simulink model "Dynamic_Simulation"  (R2019a)
settings: Solver=VariableStepAuto  StartTime=0.0  StopTime=10.0  RelTol=1e-3
values from neighbouring files (symbols this model uses):
  Car = feval(Files.Car_File)    [Run_Program.m]
settings Model: Creator=Foster  LastModifiedBy=Foster

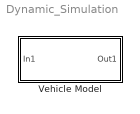
== system Dynamic_Simulation ==
  Vehicle Model : Subsystem

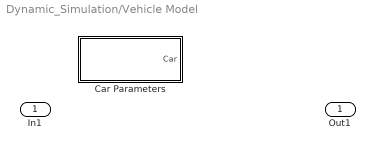
== system Dynamic_Simulation/Vehicle Model ==
  In1 : Inport
  Car Parameters : Subsystem
  Out1 : Outport

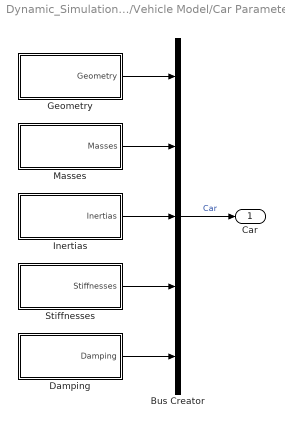
== system Dynamic_Simulation/Vehicle Model/Car Parameters ==
  Bus Creator : BusCreator  Inputs=5
  Damping : Subsystem
  Geometry : Subsystem
  Inertias : Subsystem
  Masses : Subsystem
  Stiffnesses : Subsystem
  Car : Outport
  wires:
  Geometry/1(Geometry) -> Bus Creator/1
  Masses/1(Masses) -> Bus Creator/2
  Inertias/1(Inertias) -> Bus Creator/3
  Stiffnesses/1(Stiffnesses) -> Bus Creator/4
  Damping/1(Damping) -> Bus Creator/5
  Bus Creator/1 -> Car/1  "Car"

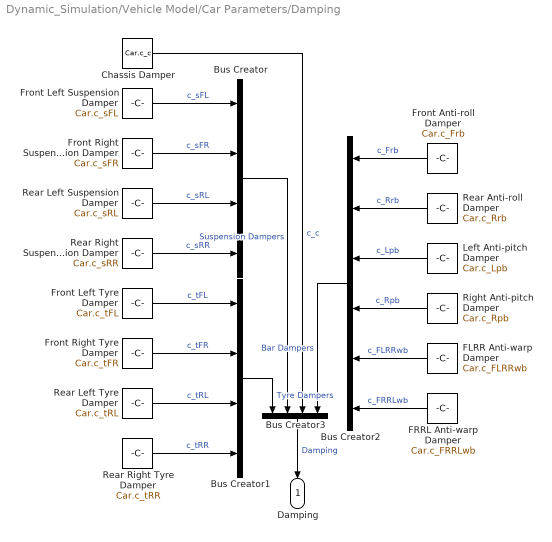
== system Dynamic_Simulation/Vehicle Model/Car Parameters/Damping ==
  Bus Creator : BusCreator  Inputs=4
  Bus Creator1 : BusCreator  Inputs=4
  Bus Creator2 : BusCreator  Inputs=6
  Bus Creator3 : BusCreator  Inputs=4
  Chassis Damper : Constant  Value=Car.c_c
  FLRR Anti-warp Damper : Constant  Value=Car.c_FLRRwb
  FRRL Anti-warp Damper : Constant  Value=Car.c_FRRLwb
  Front Anti-roll Damper : Constant  Value=Car.c_Frb
  Front Left Suspension Damper : Constant  Value=Car.c_sFL
  Front Left Tyre Damper : Constant  Value=Car.c_tFL
  Front Right Suspension Damper : Constant  Value=Car.c_sFR
  Front Right Tyre Damper : Constant  Value=Car.c_tFR
  Left Anti-pitch Damper : Constant  Value=Car.c_Lpb
  Rear Anti-roll Damper : Constant  Value=Car.c_Rrb
  Rear Left Suspension Damper : Constant  Value=Car.c_sRL
  Rear Left Tyre Damper : Constant  Value=Car.c_tRL
  Rear Right Suspension Damper : Constant  Value=Car.c_sRR
  Rear Right Tyre Damper : Constant  Value=Car.c_tRR
  Right Anti-pitch Damper : Constant  Value=Car.c_Rpb
  Damping : Outport
  wires:
  Front Left Suspension Damper/1 -> Bus Creator/1  "c_sFL"
  Front Right Suspension Damper/1 -> Bus Creator/2  "c_sFR"
  Rear Left Suspension Damper/1 -> Bus Creator/3  "c_sRL"
  Rear Right Suspension Damper/1 -> Bus Creator/4  "c_sRR"
  Front Left Tyre Damper/1 -> Bus Creator1/1  "c_tFL"
  Front Right Tyre Damper/1 -> Bus Creator1/2  "c_tFR"
  Rear Left Tyre Damper/1 -> Bus Creator1/3  "c_tRL"
  Rear Right Tyre Damper/1 -> Bus Creator1/4  "c_tRR"
  Chassis Damper/1 -> Bus Creator3/3  "c_c"
  Front Anti-roll Damper/1 -> Bus Creator2/1  "c_Frb"
  Rear Anti-roll Damper/1 -> Bus Creator2/2  "c_Rrb"
  Left Anti-pitch Damper/1 -> Bus Creator2/3  "c_Lpb"
  Right Anti-pitch Damper/1 -> Bus Creator2/4  "c_Rpb"
  FLRR Anti-warp Damper/1 -> Bus Creator2/5  "c_FLRRwb"
  FRRL Anti-warp Damper/1 -> Bus Creator2/6  "c_FRRLwb"
  Bus Creator3/1 -> Damping/1  "Damping"
  Bus Creator1/1 -> Bus Creator3/1  "Tyre Dampers"
  Bus Creator/1 -> Bus Creator3/2  "Suspension Dampers"
  Bus Creator2/1 -> Bus Creator3/4  "Bar Dampers"

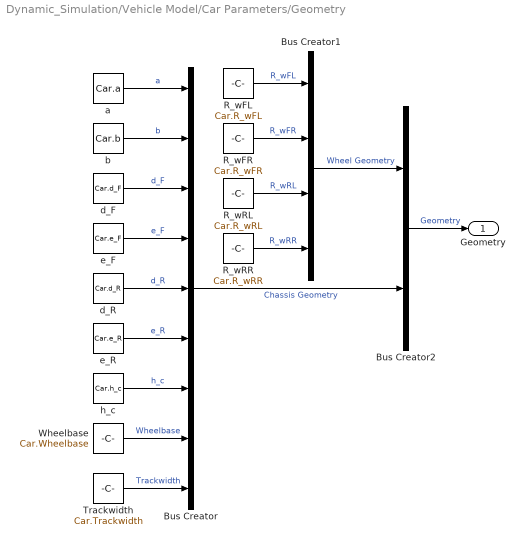
== system Dynamic_Simulation/Vehicle Model/Car Parameters/Geometry ==
  Bus Creator : BusCreator  Inputs=9
  Bus Creator1 : BusCreator  Inputs=4
  Bus Creator2 : BusCreator  Inputs=2
  R_wFL : Constant  Value=Car.R_wFL
  R_wFR : Constant  Value=Car.R_wFR
  R_wRL : Constant  Value=Car.R_wRL
  R_wRR : Constant  Value=Car.R_wRR
  Trackwidth : Constant  Value=Car.Trackwidth
  Wheelbase : Constant  Value=Car.Wheelbase
  a : Constant  Value=Car.a
  b : Constant  Value=Car.b
  d_F : Constant  Value=Car.d_F
  d_R : Constant  Value=Car.d_R
  e_F : Constant  Value=Car.e_F
  e_R : Constant  Value=Car.e_R
  h_c : Constant  Value=Car.h_c
  Geometry : Outport
  wires:
  a/1 -> Bus Creator/1  "a"
  b/1 -> Bus Creator/2  "b"
  d_F/1 -> Bus Creator/3  "d_F"
  e_F/1 -> Bus Creator/4  "e_F"
  d_R/1 -> Bus Creator/5  "d_R"
  e_R/1 -> Bus Creator/6  "e_R"
  Trackwidth/1 -> Bus Creator/9  "Trackwidth"
  Wheelbase/1 -> Bus Creator/8  "Wheelbase"
  h_c/1 -> Bus Creator/7  "h_c"
  R_wFL/1 -> Bus Creator1/1  "R_wFL"
  R_wFR/1 -> Bus Creator1/2  "R_wFR"
  R_wRL/1 -> Bus Creator1/3  "R_wRL"
  R_wRR/1 -> Bus Creator1/4  "R_wRR"
  Bus Creator/1 -> Bus Creator2/2  "Chassis Geometry"
  Bus Creator1/1 -> Bus Creator2/1  "Wheel Geometry"
  Bus Creator2/1 -> Geometry/1  "Geometry"

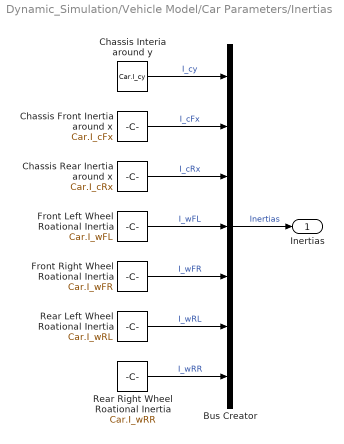
== system Dynamic_Simulation/Vehicle Model/Car Parameters/Inertias ==
  Bus Creator : BusCreator  Inputs=7
  Chassis Front Inertia around x : Constant  Value=Car.I_cFx
  Chassis Interia around y : Constant  Value=Car.I_cy
  Chassis Rear Inertia around x : Constant  Value=Car.I_cRx
  Front Left Wheel Roational Inertia : Constant  Value=Car.I_wFL
  Front Right Wheel Roational Inertia : Constant  Value=Car.I_wFR
  Rear Left Wheel Roational Inertia : Constant  Value=Car.I_wRL
  Rear Right Wheel Roational Inertia : Constant  Value=Car.I_wRR
  Inertias : Outport
  wires:
  Chassis Interia around y/1 -> Bus Creator/1  "I_cy"
  Chassis Front Inertia around x/1 -> Bus Creator/2  "I_cFx"
  Chassis Rear Inertia around x/1 -> Bus Creator/3  "I_cRx"
  Front Left Wheel Roational Inertia/1 -> Bus Creator/4  "I_wFL"
  Front Right Wheel Roational Inertia/1 -> Bus Creator/5  "I_wFR"
  Rear Left Wheel Roational Inertia/1 -> Bus Creator/6  "I_wRL"
  Rear Right Wheel Roational Inertia/1 -> Bus Creator/7  "I_wRR"
  Bus Creator/1 -> Inertias/1  "Inertias"

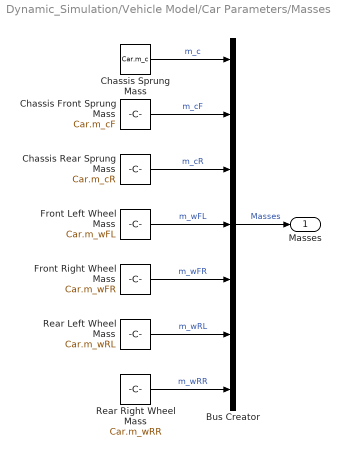
== system Dynamic_Simulation/Vehicle Model/Car Parameters/Masses ==
  Bus Creator : BusCreator  Inputs=7
  Chassis Front Sprung Mass : Constant  Value=Car.m_cF
  Chassis Rear Sprung Mass : Constant  Value=Car.m_cR
  Chassis Sprung Mass : Constant  Value=Car.m_c
  Front Left Wheel Mass : Constant  Value=Car.m_wFL
  Front Right Wheel Mass : Constant  Value=Car.m_wFR
  Rear Left Wheel Mass : Constant  Value=Car.m_wRL
  Rear Right Wheel Mass : Constant  Value=Car.m_wRR
  Masses : Outport
  wires:
  Chassis Sprung Mass/1 -> Bus Creator/1  "m_c"
  Chassis Front Sprung Mass/1 -> Bus Creator/2  "m_cF"
  Chassis Rear Sprung Mass/1 -> Bus Creator/3  "m_cR"
  Front Left Wheel Mass/1 -> Bus Creator/4  "m_wFL"
  Front Right Wheel Mass/1 -> Bus Creator/5  "m_wFR"
  Rear Left Wheel Mass/1 -> Bus Creator/6  "m_wRL"
  Rear Right Wheel Mass/1 -> Bus Creator/7  "m_wRR"
  Bus Creator/1 -> Masses/1  "Masses"

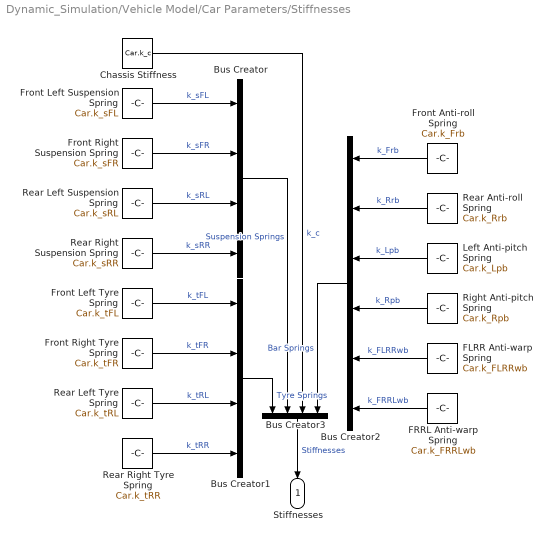
== system Dynamic_Simulation/Vehicle Model/Car Parameters/Stiffnesses ==
  Bus Creator : BusCreator  Inputs=4
  Bus Creator1 : BusCreator  Inputs=4
  Bus Creator2 : BusCreator  Inputs=6
  Bus Creator3 : BusCreator  Inputs=4
  Chassis Stiffness : Constant  Value=Car.k_c
  FLRR Anti-warp Spring : Constant  Value=Car.k_FLRRwb
  FRRL Anti-warp Spring : Constant  Value=Car.k_FRRLwb
  Front Anti-roll Spring : Constant  Value=Car.k_Frb
  Front Left Suspension Spring : Constant  Value=Car.k_sFL
  Front Left Tyre Spring : Constant  Value=Car.k_tFL
  Front Right Suspension Spring : Constant  Value=Car.k_sFR
  Front Right Tyre Spring : Constant  Value=Car.k_tFR
  Left Anti-pitch Spring : Constant  Value=Car.k_Lpb
  Rear Anti-roll Spring : Constant  Value=Car.k_Rrb
  Rear Left Suspension Spring : Constant  Value=Car.k_sRL
  Rear Left Tyre Spring : Constant  Value=Car.k_tRL
  Rear Right Suspension Spring : Constant  Value=Car.k_sRR
  Rear Right Tyre Spring : Constant  Value=Car.k_tRR
  Right Anti-pitch Spring : Constant  Value=Car.k_Rpb
  Stiffnesses : Outport
  wires:
  Front Left Suspension Spring/1 -> Bus Creator/1  "k_sFL"
  Front Right Suspension Spring/1 -> Bus Creator/2  "k_sFR"
  Rear Left Suspension Spring/1 -> Bus Creator/3  "k_sRL"
  Rear Right Suspension Spring/1 -> Bus Creator/4  "k_sRR"
  Front Left Tyre Spring/1 -> Bus Creator1/1  "k_tFL"
  Front Right Tyre Spring/1 -> Bus Creator1/2  "k_tFR"
  Rear Left Tyre Spring/1 -> Bus Creator1/3  "k_tRL"
  Rear Right Tyre Spring/1 -> Bus Creator1/4  "k_tRR"
  Chassis Stiffness/1 -> Bus Creator3/3  "k_c"
  Front Anti-roll Spring/1 -> Bus Creator2/1  "k_Frb"
  Rear Anti-roll Spring/1 -> Bus Creator2/2  "k_Rrb"
  Left Anti-pitch Spring/1 -> Bus Creator2/3  "k_Lpb"
  Right Anti-pitch Spring/1 -> Bus Creator2/4  "k_Rpb"
  FLRR Anti-warp Spring/1 -> Bus Creator2/5  "k_FLRRwb"
  FRRL Anti-warp Spring/1 -> Bus Creator2/6  "k_FRRLwb"
  Bus Creator3/1 -> Stiffnesses/1  "Stiffnesses"
  Bus Creator1/1 -> Bus Creator3/1  "Tyre Springs"
  Bus Creator/1 -> Bus Creator3/2  "Suspension Springs"
  Bus Creator2/1 -> Bus Creator3/4  "Bar Springs"
